simulink model "Flux_Controller_Type3_24a"  (R2024a)
settings: Solver=VariableStepAuto  StartTime=0.0  StopTime=10.0  RelTol=1e-3
values from neighbouring files (symbols this model uses):
  a1 = x(1)    [Model_6_6_Continuous_Weighted.m]    (also in type3_controller_function.m = 1.59505202506; type3_controller_function_fixed.m = 1.59505202506)
  a2 = x(2)    [Model_6_6_Continuous_Weighted.m]    (also in type3_controller_function.m = -0.599079946701; type3_controller_function_fixed.m = -0.599079946701)
  B_inv = [ ... (first row only)    [type3_controller_function.m]    (also in type3_controller_function_fixed.m)
  lambda_c = 0.5    [complete_test_type3.m]    (also in quick_test_type3.m; type3_controller_function.m = evalin('base', 'lambda_c'); type3_controller_function_fixed.m)
  Ts = 1e-5    (= 1e-05)    [complete_test_type3.m]    (also in generate_simulink_framework.m; quick_test_type3.m)
undefined symbols (not defined in the file or in its folder): fb_coeff_1, fb_coeff_2, l1, l2, l3
settings Model: Creator=PME406_01  LastModifiedBy=PME406_01

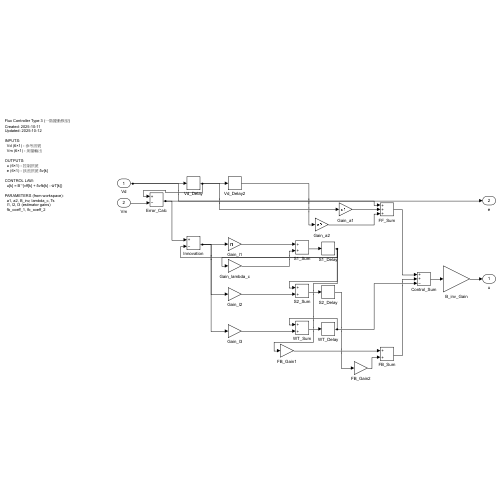
[thumbnail: Simulink's stored preview of the top-level diagram]
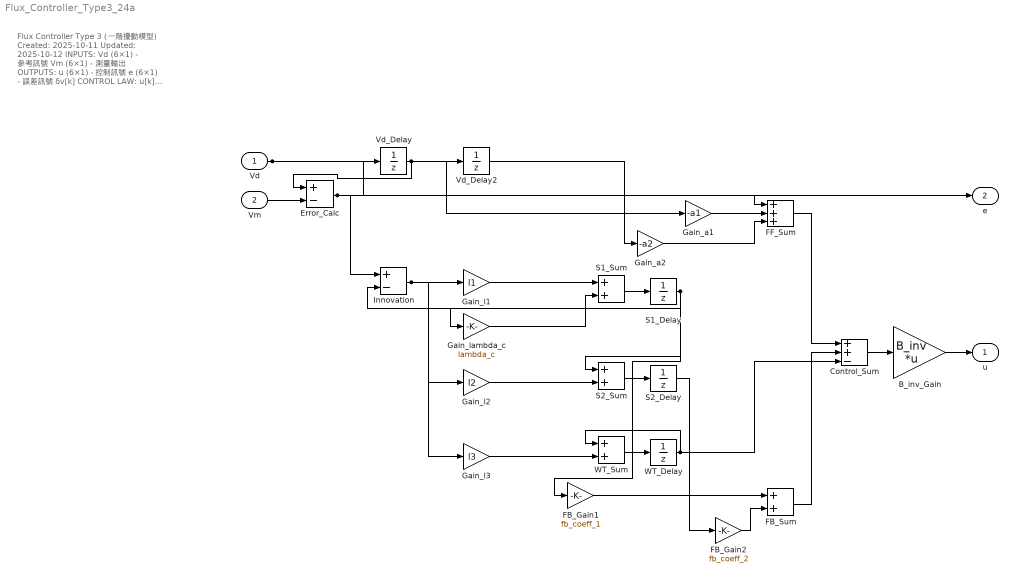
== system Flux_Controller_Type3_24a ==
  note: Flux Controller Type 3 (一階擾動模型)
      | Created: 2025-10-11
      | Updated: 2025-10-12
      |
      | INPUTS:
      |   Vd (6×1) - 參考訊號
      |   Vm (6×1) - 測量輸出
      |
      | OUTPUTS:
      |   u (6×1) - 控制訊號
      |   e (6×1) - 誤差訊號 δv[k]
      |
      | CONTROL LAW:
      |   u[k] = B⁻¹{vff[k] + δvfb[k] - ŵT[k]}
      |
      | PARAMETERS (from workspace):
      |   a1, a2, B_inv, lambda_c, Ts
      |   l1, l2, l3 (estimator gains)
      |   fb_coeff_1, fb_coeff_2
  Vd : Inport
  Vm : Inport  Port=2
  B_inv_Gain : Gain  Gain=B_inv  Multiplication=Matrix(K*u)
  Control_Sum : Sum  Inputs=++-
  Error_Calc : Sum  Inputs=+-
  FB_Gain1 : Gain  Gain=fb_coeff_1
  FB_Gain2 : Gain  Gain=fb_coeff_2
  FB_Sum : Sum
  FF_Sum : Sum  Inputs=+++
  Gain_a1 : Gain  Gain=-a1
  Gain_a2 : Gain  Gain=-a2
  Gain_l1 : Gain  Gain=l1
  Gain_l2 : Gain  Gain=l2
  Gain_l3 : Gain  Gain=l3
  Gain_lambda_c : Gain  Gain=lambda_c
  Innovation : Sum  Inputs=+-
  S1_Delay : UnitDelay  InitialCondition=zeros(6,1)  SampleTime=Ts  HasFrameUpgradeWarning=on
  S1_Sum : Sum
  S2_Delay : UnitDelay  InitialCondition=zeros(6,1)  SampleTime=Ts  HasFrameUpgradeWarning=on
  S2_Sum : Sum
  Vd_Delay : UnitDelay  SampleTime=Ts  HasFrameUpgradeWarning=on
  Vd_Delay2 : UnitDelay  SampleTime=Ts  HasFrameUpgradeWarning=on
  WT_Delay : UnitDelay  InitialCondition=zeros(6,1)  SampleTime=Ts  HasFrameUpgradeWarning=on
  WT_Sum : Sum
  u : Outport
  e : Outport  Port=2
  wires:
  Vd/1 -> Vd_Delay/1, FF_Sum/1
  Vd_Delay/1 -> Error_Calc/1, Vd_Delay2/1, Gain_a1/1
  Vm/1 -> Error_Calc/2
  Vd_Delay2/1 -> Gain_a2/1
  Gain_a1/1 -> FF_Sum/2
  Gain_a2/1 -> FF_Sum/3
  Error_Calc/1 -> Innovation/1, e/1
  Innovation/1 -> Gain_l1/1, Gain_l2/1, Gain_l3/1
  Gain_l1/1 -> S1_Sum/1
  S1_Delay/1 -> Gain_lambda_c/1, Innovation/2, S2_Sum/1, FB_Gain1/1
  Gain_lambda_c/1 -> S1_Sum/2
  S1_Sum/1 -> S1_Delay/1
  Gain_l2/1 -> S2_Sum/2
  S2_Sum/1 -> S2_Delay/1
  WT_Delay/1 -> WT_Sum/1, Control_Sum/3
  Gain_l3/1 -> WT_Sum/2
  WT_Sum/1 -> WT_Delay/1
  S2_Delay/1 -> FB_Gain2/1
  FB_Gain1/1 -> FB_Sum/1
  FB_Gain2/1 -> FB_Sum/2
  FF_Sum/1 -> Control_Sum/1
  FB_Sum/1 -> Control_Sum/2
  Control_Sum/1 -> B_inv_Gain/1
  B_inv_Gain/1 -> u/1
